simulink model "ref_disturbio"  (R2023a)
settings: Solver=VariableStepAuto  StartTime=0.0  StopTime=20.0  RelTol=1e-3
values from neighbouring files (symbols this model uses):
  Lk1 = L_a(1)    [esp_estados.m]    (also in esp_st_completo.m = 4.7046)
  Lk2 = L_a(2)    [esp_estados.m]    (also in esp_st_completo.m = 1.6662)
  Lk3 = L_a(3)    [esp_estados.m]    (also in esp_st_completo.m = -6.4214)
  Ts = 0.02    [esp_estados.m]    (also in esp_st_completo.m)
settings Model: Creator=DELL  LastModifiedBy=DELL

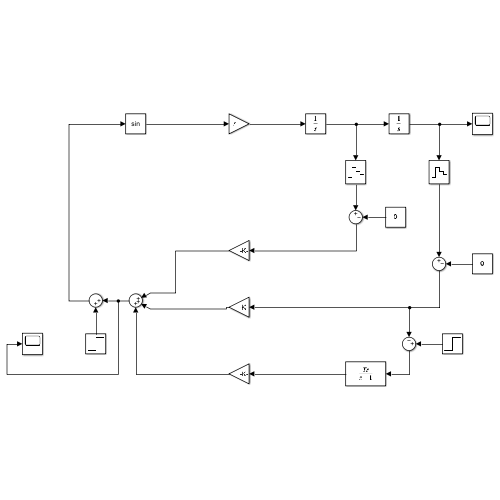
[thumbnail: Simulink's stored preview of the top-level diagram]
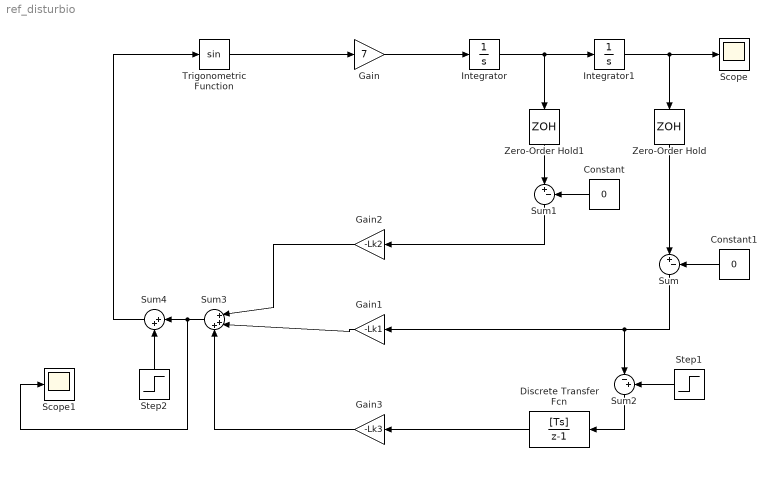
== system ref_disturbio ==
  Constant : Constant  Value=0
  Constant1 : Constant  Value=0
  Discrete Transfer Fcn : DiscreteTransferFcn  Numerator=[Ts]  Denominator=[1 -1]  SampleTime=Ts
  Gain : Gain  Gain=7
  Gain1 : Gain  Gain=-Lk1
  Gain2 : Gain  Gain=-Lk2
  Gain3 : Gain  Gain=-Lk3
  Integrator : Integrator
  Integrator1 : Integrator
  Scope : Scope
  Scope1 : Scope
  Step1 : Step  After=0.1  SampleTime=0
  Step2 : Step  Time=8  After=0.01  SampleTime=0
  Sum : Sum  Inputs=|+-
  Sum1 : Sum  Inputs=|+-
  Sum2 : Sum  Inputs=|-+
  Sum3 : Sum  Inputs=|+++
  Sum4 : Sum  Inputs=|++
  Trigonometric Function : Trigonometry
  Zero-Order Hold : ZeroOrderHold  SampleTime=Ts
  Zero-Order Hold1 : ZeroOrderHold  SampleTime=Ts
  wires:
  Trigonometric Function/1 -> Gain/1
  Gain/1 -> Integrator/1
  Integrator1/1 -> Zero-Order Hold/1, Scope/1
  Integrator/1 -> Zero-Order Hold1/1, Integrator1/1
  Zero-Order Hold/1 -> Sum/1
  Sum/1 -> Sum2/1, Gain1/1
  Zero-Order Hold1/1 -> Sum1/1
  Constant/1 -> Sum1/2
  Sum1/1 -> Gain2/1
  Sum2/1 -> Discrete Transfer Fcn/1
  Discrete Transfer Fcn/1 -> Gain3/1
  Gain3/1 -> Sum3/3
  Gain1/1 -> Sum3/2
  Gain2/1 -> Sum3/1
  Constant1/1 -> Sum/2
  Step1/1 -> Sum2/2
  Step2/1 -> Sum4/2
  Sum3/1 -> Scope1/1, Sum4/1
  Sum4/1 -> Trigonometric Function/1
